simulink model "PMStest"  (R2013a)
settings: Solver=FixedStepDiscrete  StartTime=0.0  StopTime=10.0  RelTol=1e-3
undefined symbols (not defined in the file or in its folder): ConnectedGensets, DPDesiredPower, GeneratorRatedPower, GeneratorSwbId, GensetPower, GensetPowerAvailable, HighPriorityDesiredPower, HighPriorityPower, LowPriorityDesiredPower, LowPriorityPower, nBus, SwitchToBusMapping, ThrusterConnected, ThrusterPower, ThrusterRatedPower, ThrusterSwbId
settings Model: Creator=torstein  LastModifiedBy=torstein
settings OptimizationCC: ExpressionDepthLimit=2147483647

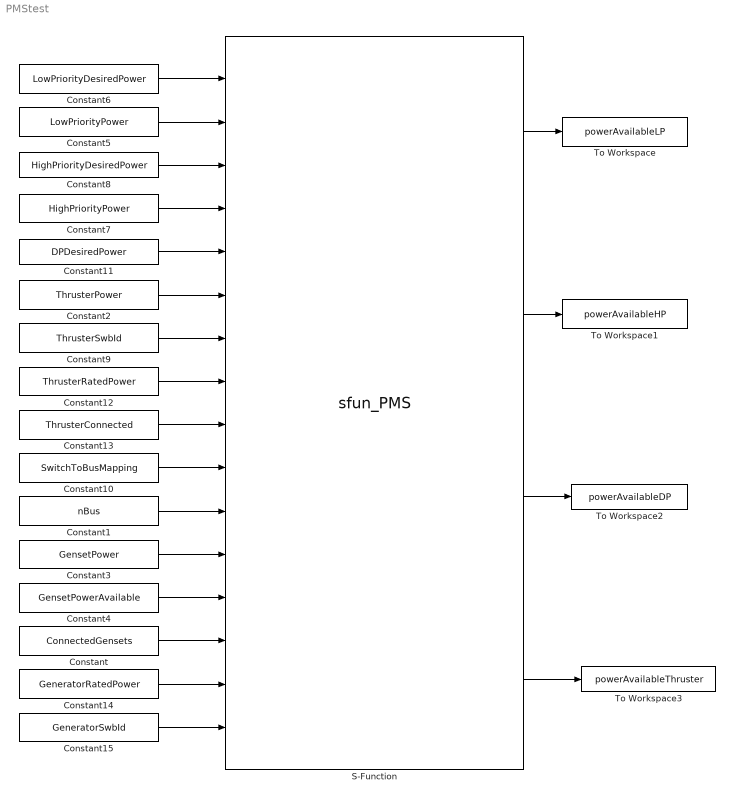
== system PMStest ==
  Constant : Constant  Value=ConnectedGensets  OutDataTypeStr=boolean
  Constant1 : Constant  Value=nBus
  Constant10 : Constant  Value=SwitchToBusMapping
  Constant11 : Constant  Value=DPDesiredPower
  Constant12 : Constant  Value=ThrusterRatedPower
  Constant13 : Constant  Value=ThrusterConnected  OutDataTypeStr=boolean
  Constant14 : Constant  Value=GeneratorRatedPower
  Constant15 : Constant  Value=GeneratorSwbId
  Constant2 : Constant  Value=ThrusterPower
  Constant3 : Constant  Value=GensetPower
  Constant4 : Constant  Value=GensetPowerAvailable
  Constant5 : Constant  Value=LowPriorityPower
  Constant6 : Constant  Value=LowPriorityDesiredPower
  Constant7 : Constant  Value=HighPriorityPower
  Constant8 : Constant  Value=HighPriorityDesiredPower
  Constant9 : Constant  Value=ThrusterSwbId
  S-Function : S-Function  FunctionName=sfun_PMS  Parameters=TSample, rampTimePowerAvaialble,FlrRestoreTime,FlrRampTime,nSwb  EnableBusSupport=off
  To Workspace : ToWorkspace  VariableName=powerAvailableLP  SampleTime=-1  SaveFormat=Timeseries
  To Workspace1 : ToWorkspace  VariableName=powerAvailableHP  SampleTime=-1  SaveFormat=Timeseries
  To Workspace2 : ToWorkspace  VariableName=powerAvailableDP  SampleTime=-1  SaveFormat=Timeseries
  To Workspace3 : ToWorkspace  VariableName=powerAvailableThruster  SampleTime=-1  SaveFormat=Timeseries
  wires:
  Constant1/1 -> S-Function/11
  Constant10/1 -> S-Function/10
  Constant11/1 -> S-Function/5
  Constant6/1 -> S-Function/1
  Constant5/1 -> S-Function/2
  Constant7/1 -> S-Function/4
  Constant8/1 -> S-Function/3
  S-Function/3 -> To Workspace2/1
  S-Function/2 -> To Workspace1/1
  S-Function/1 -> To Workspace/1
  Constant2/1 -> S-Function/6
  S-Function/4 -> To Workspace3/1
  Constant3/1 -> S-Function/12
  Constant4/1 -> S-Function/13
  Constant/1 -> S-Function/14
  Constant9/1 -> S-Function/7
  Constant13/1 -> S-Function/9
  Constant12/1 -> S-Function/8
  Constant14/1 -> S-Function/15
  Constant15/1 -> S-Function/16
